simulink model "bettersmcmodel"  (R2015a)
settings: Solver=FixedStepDiscrete  SolverMode=SingleTasking  StartTime=0.0  StopTime=2.5  RelTol=1e-3
PreLoadFcn:
  | Ts_Power=1e-6;
  | Ts_Control=100e-6;
undefined symbols (not defined in the file): D1, Delta, sigbuilder_block
libraries: powerlib x24, powerlib_meascontrol x11, re_lib x1, simulink x1
(part 1 of 2)
Description:
  | Copyright 2008-2015 The MathWorks, Inc.
settings Model: SimulationMode=accelerator  CovSFcnEnable=off  Creator=MathWorks  LastModifiedBy=teja
settings DataIOCC: SignalLoggingSaveFormat=ModelDataLogs  SignalLogging=off  DSMLogging=off
settings OptimizationCC: ExpressionDepthLimit=2147483647
settings DebuggingCC: UnderspecifiedInitializationDetection=Classic  MergeDetectMultiDrivingBlocksExec=none  SolverPrmCheckMsg=warning  FcnCallInpInsideContextMsg=UseLocalSettings  StateNameClashWarn=warning
settings GRTTargetCC: CombineOutputUpdateFcns=off  GRTInterface=on

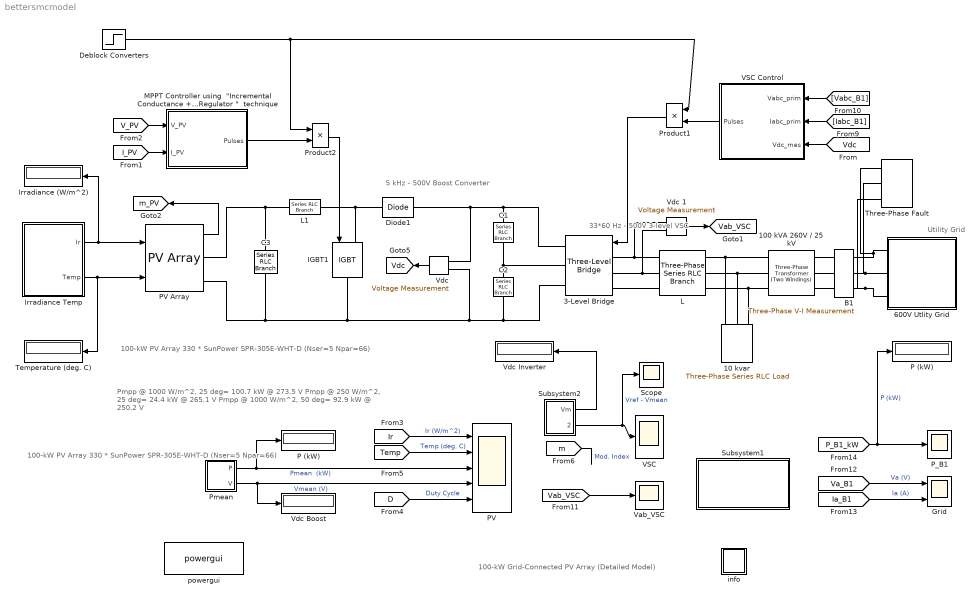
== system bettersmcmodel ==
  note: 5 kHz - 500V
      | Boost Converter
  note: 33*60 Hz - 500V
      | 3-level VSC
  note: 100-kW Grid-Connected PV Array (Detailed Model)
  note: Utility Grid
  note: Pmpp @ 1000 W/m^2, 25 deg= 100.7 kW @ 273.5 V
      | Pmpp @  250 W/m^2, 25 deg= 24.4  kW @ 265.1 V
      | Pmpp @ 1000 W/m^2, 50 deg= 92.9  kW @ 250.2 V
  note: 100-kW  PV Array
      | 330 * SunPower SPR-305E-WHT-D  (Nser=5 Npar=66)
  note: 100-kW  PV Array
      | 330 * SunPower SPR-305E-WHT-D  (Nser=5 Npar=66)
  10 kvar : powerlib/Elements/Three-Phase Series RLC Load  LConnTagsString=A|B|C  Configuration=Y (grounded)  NominalVoltage=240  NominalFrequency=60  ActivePower=10e3/100  InductivePower=0  CapacitivePower=10e3  Measurements=None  LoadType=constant Z
  100 kVA 260V / 25 kV : powerlib/Elements/Three-Phase Transformer (Two Windings)  Winding1Connection=Yg  Winding2Connection=Delta (D1)  CoreType=Three single-phase transformers  SetSaturation=off  Hysteresis=off  DataFile='hysteresis'  SetInitialFlux=off  Measurements=None  UNITS=pu  NominalPower=[100e3 , 60 ]  Winding1=[ 25e3 , 0.001 , 0.03 ]  Winding2=[ 260 , 0.001 , 0.03 ]  Rm=500  Lm=500  L0=0.5  Saturation=[ 0,0 ; 0.0024,1.2 ; 1.0,1.52 ]  InitialFluxes=[ 0.8 , -0.8 , 0.7 ]  MoreParameters=off  BreakLoop=off  DataType=off  TransfoNumber=0
  3-Level Bridge : powerlib/Power Electronics/Three-Level Bridge  Arms=3  SnubberResistance=1e6  SbubberCapacitance=inf  Device=IGBT / Diodes  Ron=0.2e-3  ForwardVoltages="[  0  0 ]"  Measurements=None
  600V Utlity Grid : Subsystem
      mask Display: image(imread('grid.jpg'))
  B1 : powerlib/Measurements/Three-Phase V-I Measurement  VoltageMeasurement=phase-to-ground  SetLabelV=on  LabelV=Vabc_B1  Vpu=off  VpuLL=off  CurrentMeasurement=yes  SetLabelI=on  LabelI=Iabc_B1  Ipu=off  Pbase=100e6  Vbase=500e3  OutputType=Magnitude  PhasorSimulation=off  PSBequivalent=0
  C1 : powerlib/Elements/Series RLC Branch  LConnTagsString=__new0  RConnTagsString=__new0  BranchType=C  Resistance=1.0  Inductance=1.0  SetiL0=off  InitialCurrent=0  Capacitance=12000e-06  Setx0=off  InitialVoltage=0  Measurements=None
  C2 : powerlib/Elements/Series RLC Branch  LConnTagsString=__new0  RConnTagsString=__new0  BranchType=C  Resistance=1.0  Inductance=1.0  SetiL0=off  InitialCurrent=0  Capacitance=12000e-06  Setx0=off  InitialVoltage=0  Measurements=None
  C3 : powerlib/Elements/Series RLC Branch  LConnTagsString=__new0  RConnTagsString=__new0  BranchType=C  Resistance=1.0  Inductance=1.0  SetiL0=off  InitialCurrent=0  Capacitance=100e-6  Setx0=off  InitialVoltage=0  Measurements=Branch voltage
  Deblock Converters : Step  Time=0.05  SampleTime=0
  Diode1 : powerlib/Power Electronics/Diode  Ron=1e-4  Lon=0  Vf=0  IC=0  UseSnubber=off  Rs=inf  Cs=inf  Measurements=off
  Grid : Scope  NumInputPorts=2
      settings: TimeRange=0.05  YMin=-15000~-2.5  YMax=15000~4  Decimation=20
  IGBT1 : powerlib/Power Electronics/IGBT  Ron=0.001  Lon=0  Vf=0  Tf=0  Tt=0  IC=0  Rs=1e5  Cs=inf  Measurements=off
  Irradiance (W/m^2) : Display
      settings: Format=bank  Decimation=1000
  Irradiance Temp : Subsystem  Tag=STV Subsys  LoadFcn=sigbuilder_block('load');  StartFcn=sigbuilder_block('start');  StopFcn=sigbuilder_block('stop');  ClipboardFcn=sigbuilder_block('clipboard');  mask(Sigbuilder block){}
      mask help: Sigbuilder GUI
      mask init:
      | if ~strcmp(get_param(bdroot(gcbh),'SimulationStatus'),'stopped') tuvar = sigbuilder_block('maskInit'); end
      settings: CopyFcn=sigbuilder_block('copy');  DeleteFcn=sigbuilder_block('delete');  ModelCloseFcn=sigbuilder_block('modelClose');  PreSaveFcn=sigbuilder_block('preSave');  PauseFcn=sigbuilder_block('pause')  ContinueFcn=sigbuilder_block('continue')  NameChangeFcn=sigbuilder_block('namechange');  OpenFcn=sigbuilder_block('open',[216.75 153.75 550.5 395.25 ]);  CloseFcn=sigbuilder_block('close');
      mask Display: plot(0,0,100,100,[10,10,40,40,10],[80,20,20,80,80],[40,10],[50,50], [40,27,10],[65,72,56],[40,25,25,10],[28,28,43,43]);
  L : powerlib/Elements/Three-Phase Series RLC Branch  LConnTagsString=A|B|C  RConnTagsString=A|B|C  BranchType=RL  Resistance=500e-6*377/50/2  Inductance=500e-6/2  Capacitance=inf  Measurements=None
  L1 : powerlib/Elements/Series RLC Branch  LConnTagsString=__new0  RConnTagsString=__new0  BranchType=RL  Resistance=0.005  Inductance=5e-3  SetiL0=off  InitialCurrent=0  Capacitance=1e-6  Setx0=off  InitialVoltage=0  Measurements=None
  "MPPT Controller using  \"Incremental Conductance + Integral Regulator \"  technique " : Subsystem  mask(Boost Control - MPPT){fc=5000, T_MPPT=200e-6, Dinit=0.5}
      mask prompts: fc "PWM switching frequency (Hz)"; T_MPPT "Time window used by MPPT control (s)"; Dinit "Initial value of duty cycle"
  P (kW) : Display
      settings: Format=bank  Decimation=2000
  "P (kW) " : Display
      settings: Format=bank  Decimation=2000
  PV : Scope  NumInputPorts=5
      settings: TimeRange=2.5  YMin=200~25~0~0~0.44  YMax=1000~50~150~400~0.52  Decimation=100
  PV Array : re_lib/Solar/PV Array  Npar=66  Nser=5  PlotType=array @ 1000 W/m2 & specified temperatures  S_vec="[ 1000  250 ]"  Temp_C_vec="[0 25 50  ]"  ModuleName=SunPower SPR-305E-WHT-D  PlotWhenSelected=off  Pm=305.226  Ncell=96  Voc=64.2  Isc=5.96  Vm=54.7  Im=5.58  beta_Voc_pc=-0.27269  alpha_Isc_pc=0.061745  beta_Voc=-0.17507  alpha_Isc=0.00368  IL=6.0092  I0=6.3014e-12  nI=0.94504  Rsh=269.5934  Rs=0.37152  BAL=on  Tc=Tc  Tfilter=5e-5
  P_B1 : Scope
      settings: TimeRange=2  YMin=50.4558  YMax=55.767  SaveName=c3  Decimation=100
  Pmean : Subsystem
  Product1 : Product  RndMeth=Zero
  Product2 : Product  RndMeth=Zero
  Scope : Scope
      settings: SaveName=c2
  Subsystem1 : Subsystem
      mask Display: disp('Open this block\nto display additional \nscopes & measurements')
  Subsystem2 : Subsystem
  "Temperature (deg. C)\t" : Display
      settings: Format=bank  Decimation=1000
  Three-Phase Fault : powerlib/Elements/Three-Phase Fault  InitialStates=0  FaultA=on  FaultB=on  FaultC=on  GroundFault=on  SwitchTimes="[1/60  5/60]"  External=off  SwitchStatus=NaN  FaultResistance=0.001  GroundResistance=0.01  SnubberResistance=1e6  SnubberCapacitance=inf  Measurements=None
  VSC : Scope
      settings: TimeRange=2  YMin=500  YMax=590  SaveName=S  Decimation=100
  VSC Control : Subsystem  mask(VSC Main Controller){nom=[ 100e3  60 ], Vnom=[ 25e3 260 ], Vnom_dc=500, RLxfo=[0.002  0.06 ], RLchoke=[2e-3  250e-6  ], K_VDCreg=[7  800], K_Ireg=[0.3 20], Ts=Ts_Control}
      mask prompts: nom "Nominal power and frequency [ Pnom(VA)  Fnom(Hz) ]:"; Vnom "Nominal primary and secondary voltages (Vrms LL) [ Vnom_prim   Vnom_sec ]:"; Vnom_dc "Nominal DC bus voltage (V):"; RLxfo "Total transformer leakage impedance (pu/Pnom) [ Rxfo  Lxf ]"; RLchoke "Choke impedance [ R(ohm) L(H) ]"; K_VDCreg "VDC regultator gains [ Kp  Ki ]:"; K_Ireg "Current regulator gains [ Kp  Ki ]:"; Ts "Sample time"
      mask init:
      | Pnom=nom(1);
      | Fnom=nom(2);
      | Vnom_prim=Vnom(1);
      | Vnom_sec=Vnom(2);
      | Zbase=Vnom_sec^2/Pnom;
      | Rtot_pu=RLxfo(1) + RLchoke(1)/Zbase;
      | Ltot_pu=RLxfo(2) + RLchoke(2)/(Zbase/(2*pi*Fnom));
      | Kp_VDCreg=K_VDCreg(1);
      | Ki_VDCreg=K_VDCreg(2);
      | Kp_Ireg=K_Ireg(1);
      | Ki_Ireg=K_Ireg(2);
      | Vdc_ref=Vnom_dc;
      | % Used to determine initial value of Boost Control (MPPT)
      | assignin('base','Vdc_ref_Inv',Vdc_ref);
  Vab_VSC : Scope
      settings: TimeRange=2  SaveName=c1  Decimation=10
  "Vdc " : powerlib/Measurements/Voltage Measurement  Tag=PoWeRsYsTeMmEaSuReMeNt  PhasorSimulation=off  OutputType=Magnitude  PSBequivalent=0
  Vdc 1 : powerlib/Measurements/Voltage Measurement  Tag=PoWeRsYsTeMmEaSuReMeNt  PhasorSimulation=off  OutputType=Magnitude  PSBequivalent=0
  Vdc Boost : Display
      settings: Format=bank  Decimation=2000
  Vdc Inverter : Display
      settings: Format=bank  Decimation=2000
  info : Subsystem
      settings: OpenFcn=showdemo(bdroot(gcb))
      mask Display: disp('?')
  powergui : powerlib/powergui  Priority=1  SimulationMode=Discrete  SolverType=Tustin/Backward Euler (TBE)  SampleTime=Ts_Power  frequency=60  SPID=off  DisableSnubberDevices=off  DisableRonSwitches=off  DisableVfSwitches=off  SwTol=0  DisplayEquations=off  Interpol=off  methode=off  Ts=0  FunctionMessages=off  echomessages=off  HookPort=off  EnableUseOfTLC=off  x0status=blocks  frequencyindice=0  Pbase=100e6  ErrMax=1e-4  Iterations=50  UnitsV=kV  UnitsW=MW  buscounter=0  RestoreLinks=warning  ResistiveCurrentMeasurement=off  Frange=[0:2:500]  Ylog=off  Xlog=on  ShowGrid=off  save=off  variable=ZData  structure=0  ZoomFFT=on  StartTime=0.0  cycles=1  DisplayStyle=1  fundamental=60  FreqAxis=off  MaxFrequency=1000  frequencyindicesteady=1  RmsSteady=1  display=off
  tag scope: Vab_VSC=global, Vdc=global, m_PV=global
  wires:
  "Vdc "/1 -> [Vdc]
  Product2/1 -> IGBT1/1
  "MPPT Controller using  \"Incremental Conductance + Integral Regulator \"  technique "/1(Pulses) -> Product2/2
  Deblock Converters/1 -> Product2/1, Product1/1
  [Vabc_B1] -> VSC Control/1(Vabc_prim)
  [Iabc_B1] -> VSC Control/2(Iabc_prim)
  [Vdc] -> VSC Control/3(Vdc_mes)
  VSC Control/1(Pulses) -> Product1/2
  Product1/1 -> 3-Level Bridge/1
  [I_PV] -> "MPPT Controller using  \"Incremental Conductance + Integral Regulator \"  technique "/2(I_PV)
  [V_PV] -> "MPPT Controller using  \"Incremental Conductance + Integral Regulator \"  technique "/1(V_PV)
  Pmean/1(P) -> "P (kW) "/1, PV/3  "Pmean  (kW)"
  [m] -> ?  "Mod. Index"
  Vdc 1/1 -> [Vab_VSC]
  [Vab_VSC] -> Vab_VSC/1
  [Ia_B1] -> Grid/2  "Ia (A)"
  [Va_B1] -> Grid/1  "Va (V)"
  [P_B1_kW] -> P_B1/1, P (kW)/1  "P (kW)"
  Pmean/2(V) -> Vdc Boost/1, PV/4  "Vmean (V)"
  Subsystem2/2(VrVm) -> Scope/1, VSC/1  "Vref - Vmean"
  Subsystem2/1(Vm) -> Vdc Inverter/1
  PV Array/1 -> [m_PV]
  Irradiance Temp/1(Ir) -> PV Array/1, Irradiance (W/m^2)/1
  Irradiance Temp/2(Temp) -> PV Array/2, "Temperature (deg. C)\t"/1
  [D] -> PV/5  "Duty Cycle"
  [Temp] -> PV/2  "Temp (deg. C)"
  [Ir] -> PV/1  "Ir (W/m^2)"
  connections:
  3-Level Bridge/RConn1 -- Diode1/RConn1 -- "Vdc "/LConn1 -- C1/LConn1
  L1/RConn1 -- Diode1/LConn1 -- IGBT1/LConn1
  3-Level Bridge/RConn3 -- C2/RConn1 -- "Vdc "/LConn2 -- IGBT1/RConn1 -- PV Array/RConn2 -- C3/RConn1
  3-Level Bridge/LConn1 -- L/LConn1 -- Vdc 1/LConn1
  3-Level Bridge/LConn2 -- L/LConn2 -- Vdc 1/LConn2
  3-Level Bridge/LConn3 -- L/LConn3
  L/RConn1 -- 100 kVA 260V / 25 kV/RConn1 -- 10 kvar/LConn1
  L/RConn2 -- 100 kVA 260V / 25 kV/RConn2 -- 10 kvar/LConn2
  L/RConn3 -- 100 kVA 260V / 25 kV/RConn3 -- 10 kvar/LConn3
  B1/LConn1 -- 100 kVA 260V / 25 kV/LConn1
  B1/LConn2 -- 100 kVA 260V / 25 kV/LConn2
  B1/LConn3 -- 100 kVA 260V / 25 kV/LConn3
  C2/LConn1 -- C1/RConn1 -- 3-Level Bridge/RConn2
  C3/LConn1 -- PV Array/RConn1 -- L1/LConn1
  B1/RConn2 -- 600V Utlity Grid/LConn2 -- Three-Phase Fault/LConn2
  B1/RConn1 -- Three-Phase Fault/LConn1 -- 600V Utlity Grid/LConn1
  B1/RConn3 -- 600V Utlity Grid/LConn3 -- Three-Phase Fault/LConn3

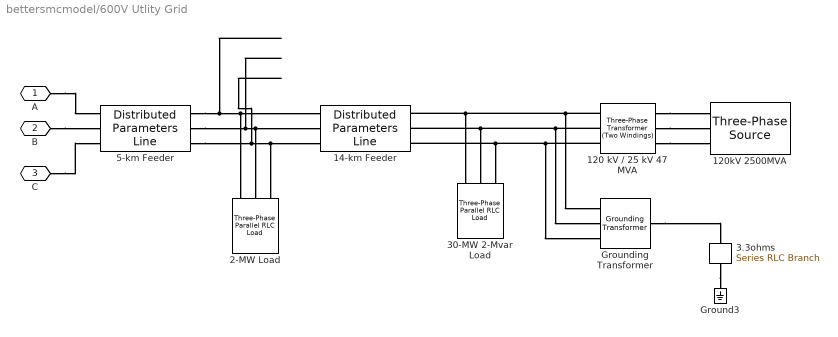
== system bettersmcmodel/600V Utlity Grid ==
  120 kV / 25 kV 47 MVA : powerlib/Elements/Three-Phase Transformer (Two Windings)  Winding1Connection=Yg  Winding2Connection=Delta (D1)  CoreType=Three single-phase transformers  SetSaturation=off  Hysteresis=off  DataFile='basic_model'  SetInitialFlux=off  Measurements=None  UNITS=pu  NominalPower=[47e6 60 ]  Winding1="[ 120e3  0.08/30   0.08 ]"  Winding2="[ 25e3  0.08/30  0.08]"  Rm=500  Lm=500  L0=0.5  Saturation="[ 0,0  ;  0.005,1.2  ;  1.0,1.4 ]"  InitialFluxes=[ 0.8 , -0.8 , 0.7 ]  MoreParameters=off  BreakLoop=off  DataType=off  TransfoNumber=0
  120kV 2500MVA : powerlib/Electrical Sources/Three-Phase Source  Voltage=120e3  PhaseAngle=0  Frequency=60  InternalConnection=Yg  SpecifyImpedance=on  Resistance=0.8929  Inductance=16.58e-3  ShortCircuitLevel=2500e6  BaseVoltage=120e3  XRratio=7  BusType=swing  Pref=0  Qref=0  Qmin=-inf  Qmax=inf
  14-km Feeder : powerlib/Elements/Distributed Parameters Line  Phases=3  Frequency=60  Resistance=[0.1153 0.413]  Inductance=[1.05e-3 3.32e-3]  Capacitance=[11.33e-009 5.01e-009]  Length=14  x1=[-5.8e-05 -2.78846572041482e-09 0 0;-5.7e-05 -2.78728594542614e-09 0 0;-5.6e-05 -2.78610577430196e-09 0 0;-5.5e-05 -2.78492520721002e-09 0 0;-5.4e-05 -2.7837442443181e-09 0 0;-5.3e-05 -2.78256288579404e-09 0 0;-5.2e-05 -2.78138113180574e-09 0 0;-5.1e-05 -2.78019898252115e-09 0 0;-5e-05 -2.77901643810828e-09 0 0;-4.9e-05 -2.7778334987352e-09 -3790.91356131619 -24061.331995883;-4.8e-05 -2.77665016457003e-09 -3781.84238368431 -24062.7594267666;-4.7e-05 -2.77546643578094e-09 -3772.77066856828 -24064.1834377954;-4.6e-05 -2.77428231253618e-09 -3763.6984172574 -24065.6040287671;-4.5e-05 -2.77309779500403e-09 -3754.62563104105 -24067.0211994797;-4.4e-05 -2.77191288335284e-09 -3745.55231120865 -24068.4349497319;-4.3e-05 -2.77072757775101e-09 -3736.47845904974 -24069.8452793227;-4.2e-05 -2.76954187836699e-09 -3727.40407585391 -24071.2521880517;-4.1e-05 -2.76835578536932e-09 -3718.32916291083 -24072.6556757189;-4e-05 -2.76716929892654e-09 -3709.25372151026 -24074.0557421249;-3.9e-05 -2.7659824192073e-09 -3700.177752942 -24075.4523870707;-3.8e-05 -2.76479514638027e-09 -3691.10125849597 -24076.8456103578;-3.7e-05 -2.76360748061418e-09 -3682.02423946214 -24078.2354117881;-3.6e-05 -2.76241942207785e-09 -3672.94669713054 -24079.6217911643;-3.5e-05 -2.7612309709401e-09 -3663.8686327913 -24081.0047482891;-3.4e-05 -2.76004212736986e-09 -3654.79004773462 -24082.3842829662;-3.3e-05 -2.75885289153607e-09 -3645.71094325077 -24083.7603949993;-3.2e-05 -2.75766326360776e-09 -3636.63132063009 -24085.133084193;-3.1e-05 -2.756473243754e-09 -3627.55118116299 -24086.5023503521;-3e-05 -2.75528283214392e-09 -3618.47052613997 -24087.8681932821;-2.9e-05 -2.7540920289467e-09 -3609.38935685159 -24089.2306127888;-2.8e-05 -2.75290083433159e-09 -3600.30767458848 -24090.5896086786;-2.7e-05 -2.75170924846787e-09 -3591.22548064137 -24091.9451807584;-2.6e-05 -2.75051727152489e-09 -3582.14277630102 -24093.2973288354;-2.5e-05 -2.74932490367208e-09 -3573.05956285829 -24094.6460527176;-2.4e-05 -2.74813214507888e-09 -3563.97584160412 -24095.9913522133;-2.3e-05 -2.74693899591481e-09 -3554.8916138295 -24097.3332271312;-2.2e-05 -2.74574545634945e-09 -3545.80688082549 -24098.6716772806;-2.1e-05 -2.74455152655243e-09 -3536.72164388326 -24100.0067024713;-2e-05 -2.74335720669342e-09 -3527.635904294 -24101.3383025136;-1.9e-05 -2.74216249694218e-09 -3518.54966334901 -24102.6664772183;-1.8e-05 -2.74096739746849e-09 -3509.46292233964 -24103.9912263965;-1.7e-05 -2.7397719084422e-09 -3500.37568255732 -24105.31254986;-1.6e-05 -2.73857603003323e-09 -3491.28794529356 -24106.630447421;-1.5e-05 -2.73737976241153e-09 -3482.19971183991 -24107.9449188921;-1.4e-05 -2.73618310574711e-09 -3473.11098348803 -24109.2559640867;-1.3e-05 -2.73498606021005e-09 -3464.02176152962 -24110.5635828183;-1.2e-05 -2.73378862597048e-09 -3454.93204725646 -24111.8677749011;-1.1e-05 -2.73259080319858e-09 -3445.84184196041 -24113.1685401498;-1e-05 -2.73139259206458e-09 -3436.75114693339 -24114.4658783794;-9e-06 -2.73019399273878e-09 -3427.65996346738 -24115.7597894057;-8e-06 -2.72899500539153e-09 -3418.56829285445 -24117.0502730447;-7e-06 -2.72779563019322e-09 -3409.47613638673 -24118.337329113;-6e-06 -2.72659586731433e-09 -3400.38349535641 -24119.6209574276;-5e-06 -2.72539571692535e-09 -3391.29037105576 -24120.9011578063;-4e-06 -2.72419517919685e-09 -3382.19676477711 -24122.1779300669;-3e-06 -2.72299425429947e-09 -3373.10267781288 -24123.4512740281;-2e-06 -2.72179294240388e-09 -3364.00811145553 -24124.7211895088;-1e-06 -2.72059124368081e-09 -3354.91306699761 -24125.9876763287]  x2=[-5.8e-05 -2.84238474455657e-09 0 0;-5.7e-05 -2.8410909495707e-09 0 0;-5.6e-05 -2.83979675080246e-09 0 0;-5.5e-05 -2.83850214843576e-09 0 0;-5.4e-05 -2.8372071426546e-09 0 0;-5.3e-05 -2.83591173364303e-09 0 0;-5.2e-05 -2.83461592158516e-09 0 0;-5.1e-05 -2.83331970666515e-09 0 0;-5e-05 -2.83202308906722e-09 0 0;-4.9e-05 -2.83072606897565e-09 -3379.44571071679 -24244.0324946947;-4.8e-05 -2.82942864657478e-09 -3370.30568586053 -24245.3047928739;-4.7e-05 -2.828130822049e-09 -3361.16518200868 -24246.5736452545;-4.6e-05 -2.82683259558275e-09 -3352.02420046029 -24247.8390516562;-4.5e-05 -2.82553396736055e-09 -3342.8827425145 -24249.1010118993;-4.4e-05 -2.82423493756696e-09 -3333.74080947053 -24250.3595258043;-4.3e-05 -2.8229355063866e-09 -3324.59840262764 -24251.6145931924;-4.2e-05 -2.82163567400415e-09 -3315.45552328517 -24252.8662138852;-4.1e-05 -2.82033544060434e-09 -3306.31217274253 -24254.1143877048;-4e-05 -2.81903480637196e-09 -3297.1683522992 -24255.3591144739;-3.9e-05 -2.81773377149187e-09 -3288.02406325471 -24256.6003940155;-3.8e-05 -2.81643233614897e-09 -3278.87930690867 -24257.8382261532;-3.7e-05 -2.81513050052823e-09 -3269.73408456076 -24259.0726107112;-3.6e-05 -2.81382826481466e-09 -3260.58839751071 -24260.3035475139;-3.5e-05 -2.81252562919334e-09 -3251.44224705834 -24261.5310363864;-3.4e-05 -2.8112225938494e-09 -3242.29563450351 -24262.7550771543;-3.3e-05 -2.80991915896804e-09 -3233.14856114616 -24263.9756696435;-3.2e-05 -2.8086153247345e-09 -3224.0010282863 -24265.1928136808;-3.1e-05 -2.80731109133408e-09 -3214.85303722399 -24266.4065090929;-3e-05 -2.80600645895215e-09 -3205.70458925937 -24267.6167557075;-2.9e-05 -2.80470142777413e-09 -3196.55568569263 -24268.8235533526;-2.8e-05 -2.80339599798548e-09 -3187.40632782404 -24270.0269018566;-2.7e-05 -2.80209016977174e-09 -3178.25651695392 -24271.2268010485;-2.6e-05 -2.8007839433185e-09 -3169.10625438268 -24272.4232507578;-2.5e-05 -2.79947731881139e-09 -3159.95554141076 -24273.6162508144;-2.4e-05 -2.79817029643613e-09 -3150.80437933868 -24274.8058010489;-2.3e-05 -2.79686287637846e-09 -3141.65276946704 -24275.991901292;-2.2e-05 -2.7955550588242e-09 -3132.50071309647 -24277.1745513753;-2.1e-05 -2.79424684395923e-09 -3123.34821152769 -24278.3537511307;-2e-05 -2.79293823196946e-09 -3114.19526606148 -24279.5295003906;-1.9e-05 -2.79162922304088e-09 -3105.04187799866 -24280.7017989878;-1.8e-05 -2.79031981735953e-09 -3095.88804864015 -24281.8706467558;-1.7e-05 -2.7890100151115e-09 -3086.7337792869 -24283.0360435285;-1.6e-05 -2.78769981648295e-09 -3077.57907123994 -24284.1979891402;-1.5e-05 -2.78638922166009e-09 -3068.42392580036 -24285.3564834258;-1.4e-05 -2.78507823082918e-09 -3059.26834426931 -24286.5115262206;-1.3e-05 -2.78376684417654e-09 -3050.112327948 -24287.6631173605;-1.2e-05 -2.78245506188854e-09 -3040.9558781377 -24288.8112566818;-1.1e-05 -2.78114288415163e-09 -3031.79899613976 -24289.9559440214;-1e-05 -2.7798303111523e-09 -3022.64168325557 -24291.0971792165;-9e-06 -2.77851734307708e-09 -3013.48394078658 -24292.234962105;-8e-06 -2.77720398011258e-09 -3004.32577003432 -24293.3692925251;-7e-06 -2.77589022244546e-09 -2995.16717230036 -24294.5001703157;-6e-06 -2.77457607026243e-09 -2986.00814888636 -24295.627595316;-5e-06 -2.77326152375026e-09 -2976.848701094 -24296.7515673657;-4e-06 -2.77194658309578e-09 -2967.68883022505 -24297.8720863053;-3e-06 -2.77063124848587e-09 -2958.52853758134 -24298.9891519753;-2e-06 -2.76931552010748e-09 -2949.36782446474 -24300.102764217;-1e-06 -2.76799939814759e-09 -2940.20669217719 -24301.2129228722]  x3=[-5.8e-05 -2.00460551784577e-11 0 0;-5.7e-05 -2.00435398524558e-11 0 0;-5.6e-05 -2.00410216778199e-11 0 0;-5.5e-05 -2.00385006549079e-11 0 0;-5.4e-05 -2.0035976784078e-11 0 0;-5.3e-05 -2.00334500656889e-11 0 0;-5.2e-05 -2.00309205000999e-11 0 0;-5.1e-05 -2.00283880876703e-11 0 0;-5e-05 -2.00258528287601e-11 0 0;-4.9e-05 -2.00233147237296e-11 -23.5492221256945 -155.70495879038;-4.8e-05 -2.00207737729395e-11 -23.4905210670905 -155.713825573184;-4.7e-05 -2.0018229976751e-11 -23.4318166699595 -155.72267022558;-4.6e-05 -2.00156833355256e-11 -23.3731089426448 -155.731492746312;-4.5e-05 -2.00131338496251e-11 -23.3143978934901 -155.740293134126;-4.4e-05 -2.00105815194121e-11 -23.2556835308395 -155.74907138777;-4.3e-05 -2.00080263452491e-11 -23.1969658630377 -155.757827505999;-4.2e-05 -2.00054683274993e-11 -23.1382448984296 -155.766561487566;-4.1e-05 -2.00029074665264e-11 -23.0795206453609 -155.775273331231;-4e-05 -2.00003437626942e-11 -23.0207931121777 -155.783963035756;-3.9e-05 -1.99977772163671e-11 -22.9620623072263 -155.792630599905;-3.8e-05 -1.99952078279099e-11 -22.9033282388538 -155.801276022447;-3.7e-05 -1.99926355976878e-11 -22.8445909154075 -155.809899302153;-3.6e-05 -1.99900605260662e-11 -22.7858503452354 -155.818500437797;-3.5e-05 -1.99874826134112e-11 -22.7271065366859 -155.827079428158;-3.4e-05 -1.99849018600892e-11 -22.6683594981076 -155.835636272015;-3.3e-05 -1.9982318266467e-11 -22.6096092378499 -155.844170968154;-3.2e-05 -1.99797318329117e-11 -22.5508557642625 -155.852683515359;-3.1e-05 -1.99771425597909e-11 -22.4920990856955 -155.861173912423;-3e-05 -1.99745504474726e-11 -22.4333392104997 -155.869642158138;-2.9e-05 -1.99719554963252e-11 -22.3745761470261 -155.878088251301;-2.8e-05 -1.99693577067176e-11 -22.3158099036262 -155.886512190711;-2.7e-05 -1.99667570790189e-11 -22.257040488652 -155.894913975171;-2.6e-05 -1.99641536135987e-11 -22.1982679104561 -155.903293603487;-2.5e-05 -1.9961547310827e-11 -22.1394921773911 -155.911651074468;-2.4e-05 -1.99589381710743e-11 -22.0807132978106 -155.919986386926;-2.3e-05 -1.99563261947114e-11 -22.0219312800683 -155.928299539677;-2.2e-05 -1.99537113821094e-11 -21.9631461325185 -155.936590531539;-2.1e-05 -1.99510937336401e-11 -21.9043578635158 -155.944859361334;-2e-05 -1.99484732496754e-11 -21.8455664814153 -155.953106027887;-1.9e-05 -1.99458499305877e-11 -21.7867719945726 -155.961330530025;-1.8e-05 -1.994322377675e-11 -21.7279744113437 -155.96953286658;-1.7e-05 -1.99405947885354e-11 -21.6691737400851 -155.977713036386;-1.6e-05 -1.99379629663175e-11 -21.6103699891537 -155.985871038281;-1.5e-05 -1.99353283104705e-11 -21.5515631669067 -155.994006871104;-1.4e-05 -1.99326908213687e-11 -21.492753281702 -156.0021205337;-1.3e-05 -1.99300504993871e-11 -21.4339403418977 -156.010212024916;-1.2e-05 -1.99274073449007e-11 -21.3751243558524 -156.018281343601;-1.1e-05 -1.99247613582854e-11 -21.3163053319253 -156.026328488609;-1e-05 -1.99221125399172e-11 -21.2574832784758 -156.034353458796;-9e-06 -1.99194608901724e-11 -21.1986582038639 -156.042356253022;-8e-06 -1.9916806409428e-11 -21.1398301164499 -156.050336870149;-7e-06 -1.99141490980613e-11 -21.0809990245945 -156.058295309043;-6e-06 -1.99114889564498e-11 -21.0221649366591 -156.066231568572;-5e-06 -1.99088259849717e-11 -20.9633278610051 -156.07414564761;-4e-06 -1.99061601840055e-11 -20.9044878059948 -156.08203754503;-3e-06 -1.99034915539299e-11 -20.8456447799906 -156.089907259713;-2e-06 -1.99008200951243e-11 -20.7867987913553 -156.097754790538;-1e-06 -1.98981458079683e-11 -20.7279498484524 -156.105580136391]  x4=[-5.8e-05 1.32145554520631e-11 0 0;-5.7e-05 1.32154032927262e-11 0 0;-5.6e-05 1.32162492551857e-11 0 0;-5.5e-05 1.32170933393215e-11 0 0;-5.4e-05 1.32179355450135e-11 0 0;-5.3e-05 1.32187758721422e-11 0 0;-5.2e-05 1.32196143205879e-11 0 0;-5.1e-05 1.32204508902317e-11 0 0;-5e-05 1.32212855809546e-11 0 0;-4.9e-05 1.32221183926379e-11 -1.35163069912945 -2.12916945889706;-4.8e-05 1.32229493251633e-11 -1.35082792512439 -2.12967886035273;-4.7e-05 1.32237783784127e-11 -1.35002495913656 -2.13018795913354;-4.6e-05 1.32246055522683e-11 -1.34922180128007 -2.13069675516714;-4.5e-05 1.32254308466125e-11 -1.34841845166907 -2.13120524838121;-4.4e-05 1.32262542613281e-11 -1.34761491041774 -2.13171343870348;-4.3e-05 1.32270757962979e-11 -1.34681117764028 -2.13222132606173;-4.2e-05 1.32278954514053e-11 -1.34600725345092 -2.13272891038378;-4.1e-05 1.32287132265338e-11 -1.3452031379639 -2.13323619159748;-4e-05 1.3229529121567e-11 -1.34439883129352 -2.13374316963075;-3.9e-05 1.32303431363892e-11 -1.34359433355408 -2.13424984441153;-3.8e-05 1.32311552708845e-11 -1.34278964485992 -2.13475621586781;-3.7e-05 1.32319655249376e-11 -1.34198476532541 -2.13526228392762;-3.6e-05 1.32327738984333e-11 -1.34117969506494 -2.13576804851904;-3.5e-05 1.32335803912567e-11 -1.34037443419291 -2.13627350957019;-3.4e-05 1.32343850032932e-11 -1.33956898282379 -2.13677866700923;-3.3e-05 1.32351877344284e-11 -1.33876334107205 -2.13728352076437;-3.2e-05 1.32359885845483e-11 -1.33795750905217 -2.13778807076386;-3.1e-05 1.3236787553539e-11 -1.33715148687869 -2.13829231693598;-3e-05 1.32375846412871e-11 -1.33634527466617 -2.13879625920908;-2.9e-05 1.32383798476791e-11 -1.33553887252918 -2.13929989751153;-2.8e-05 1.32391731726021e-11 -1.33473228058233 -2.13980323177176;-2.7e-05 1.32399646159433e-11 -1.33392549894026 -2.14030626191823;-2.6e-05 1.32407541775903e-11 -1.33311852771763 -2.14080898787944;-2.5e-05 1.32415418574309e-11 -1.33231136702912 -2.14131140958395;-2.4e-05 1.3242327655353e-11 -1.33150401698945 -2.14181352696036;-2.3e-05 1.3243111571245e-11 -1.33069647771337 -2.1423153399373;-2.2e-05 1.32438936049956e-11 -1.32988874931564 -2.14281684844345;-2.1e-05 1.32446737564935e-11 -1.32908083191107 -2.14331805240754;-2e-05 1.32454520256279e-11 -1.32827272561446 -2.14381895175833;-1.9e-05 1.32462284122881e-11 -1.32746443054068 -2.14431954642464;-1.8e-05 1.32470029163639e-11 -1.3266559468046 -2.14481983633532;-1.7e-05 1.32477755377452e-11 -1.32584727452112 -2.14531982141927;-1.6e-05 1.3248546276322e-11 -1.32503841380517 -2.14581950160543;-1.5e-05 1.3249315131985e-11 -1.32422936477172 -2.14631887682278;-1.4e-05 1.32500821046249e-11 -1.32342012753574 -2.14681794700035;-1.3e-05 1.32508471941325e-11 -1.32261070221225 -2.14731671206722;-1.2e-05 1.32516104003993e-11 -1.32180108891627 -2.14781517195249;-1.1e-05 1.32523717233167e-11 -1.32099128776289 -2.14831332658532;-1e-05 1.32531311627765e-11 -1.32018129886718 -2.14881117589492;-9e-06 1.32538887186708e-11 -1.31937112234427 -2.14930871981053;-8e-06 1.3254644390892e-11 -1.3185607583093 -2.14980595826144;-7e-06 1.32553981793326e-11 -1.31775020687744 -2.15030289117698;-6e-06 1.32561500838854e-11 -1.31693946816388 -2.15079951848652;-5e-06 1.32569001044438e-11 -1.31612854228386 -2.15129584011948;-4e-06 1.32576482409009e-11 -1.31531742935262 -2.15179185600533;-3e-06 1.32583944931506e-11 -1.31450612948544 -2.15228756607356;-2e-06 1.32591388610867e-11 -1.31369464279762 -2.15278297025373;-1e-06 1.32598813446035e-11 -1.31288296940449 -2.15327806847543]  x5=5.70973484498186e-05  V1=ones(3,3)  V2=ones(3,3)  I1=ones(3,3)  I2=ones(3,3)  nHarmo=1  Measurements=None
  2-MW Load : powerlib/Elements/Three-Phase Parallel RLC Load  LConnTagsString=A|B|C  Configuration=Y (grounded)  NominalVoltage=25e3  NominalFrequency=60  ActivePower=2e6  InductivePower=0  CapacitivePower=0  Measurements=None  LoadType=constant Z
  "3.3ohms " : powerlib/Elements/Series RLC Branch  LConnTagsString=__new0  RConnTagsString=__new0  BranchType=R  Resistance=3.3  Inductance=[]  SetiL0=off  InitialCurrent=0  Capacitance=[]  Setx0=off  InitialVoltage=0  Measurements=None
  30-MW 2-Mvar Load : powerlib/Elements/Three-Phase Parallel RLC Load  LConnTagsString=A|B|C  Configuration=Y (grounded)  NominalVoltage=25e3  NominalFrequency=60  ActivePower=30e6  InductivePower=2e6  CapacitivePower=0  Measurements=None  LoadType=constant Z
  5-km Feeder : powerlib/Elements/Distributed Parameters Line  Phases=3  Frequency=60  Resistance=[0.1153 0.413]  Inductance=[1.05e-3 3.32e-3]  Capacitance=[11.33e-009 5.01e-009]  Length=5  x1=[-2.1e-05 -2.68247201757925e-09 -3537.40246322704 -24101.3113737726;-2e-05 -2.68128874623808e-09 -3528.31623173992 -24102.643230385;-1.9e-05 -2.68010509382599e-09 -3519.22949880037 -24103.9716614744;-1.8e-05 -2.67892106051119e-09 -3510.14226569983 -24105.2966668517;-1.7e-05 -2.67773664646197e-09 -3501.0545337298 -24106.6182463289;-1.6e-05 -2.67655185184664e-09 -3491.96630418183 -24107.9363997179;-1.5e-05 -2.67536667683361e-09 -3482.87757834758 -24109.2511268316;-1.4e-05 -2.67418112159131e-09 -3473.78835751874 -24110.5624274829;-1.3e-05 -2.67299518628823e-09 -3464.69864298711 -24111.8703014857;-1.2e-05 -2.67180887109293e-09 -3455.60843604454 -24113.174748654;-1.1e-05 -2.670622176174e-09 -3446.51773798294 -24114.4757688023;-1e-05 -2.66943510170009e-09 -3437.4265500943 -24115.7733617459;-9e-06 -2.66824764783993e-09 -3428.3348736707 -24117.0675273002;-8e-06 -2.66705981476227e-09 -3419.24271000425 -24118.3582652814;-7e-06 -2.66587160263593e-09 -3410.15006038715 -24119.645575506;-6e-06 -2.66468301162978e-09 -3401.05692611168 -24120.9294577911;-5e-06 -2.66349404191275e-09 -3391.96330847017 -24122.2099119541;-4e-06 -2.66230469365381e-09 -3382.86920875503 -24123.4869378132;-3e-06 -2.661114967022e-09 -3373.77462825873 -24124.7605351867;-2e-06 -2.65992486218641e-09 -3364.67956827382 -24126.0307038938;-1e-06 -2.65873437931618e-09 -3355.5840300929 -24127.2974437538]  x2=[-2.1e-05 -2.74455152655243e-09 -3536.72164388326 -24100.0067024713;-2e-05 -2.74335720669342e-09 -3527.635904294 -24101.3383025136;-1.9e-05 -2.74216249694218e-09 -3518.54966334901 -24102.6664772183;-1.8e-05 -2.74096739746849e-09 -3509.46292233964 -24103.9912263965;-1.7e-05 -2.7397719084422e-09 -3500.37568255732 -24105.31254986;-1.6e-05 -2.73857603003323e-09 -3491.28794529356 -24106.630447421;-1.5e-05 -2.73737976241153e-09 -3482.19971183991 -24107.9449188921;-1.4e-05 -2.73618310574711e-09 -3473.11098348803 -24109.2559640867;-1.3e-05 -2.73498606021005e-09 -3464.02176152962 -24110.5635828183;-1.2e-05 -2.73378862597048e-09 -3454.93204725646 -24111.8677749011;-1.1e-05 -2.73259080319858e-09 -3445.84184196041 -24113.1685401498;-1e-05 -2.73139259206458e-09 -3436.75114693339 -24114.4658783794;-9e-06 -2.73019399273878e-09 -3427.65996346738 -24115.7597894057;-8e-06 -2.72899500539153e-09 -3418.56829285445 -24117.0502730447;-7e-06 -2.72779563019322e-09 -3409.47613638673 -24118.337329113;-6e-06 -2.72659586731433e-09 -3400.38349535641 -24119.6209574276;-5e-06 -2.72539571692535e-09 -3391.29037105576 -24120.9011578063;-4e-06 -2.72419517919685e-09 -3382.19676477711 -24122.1779300669;-3e-06 -2.72299425429947e-09 -3373.10267781288 -24123.4512740281;-2e-06 -2.72179294240388e-09 -3364.00811145553 -24124.7211895088;-1e-06 -2.72059124368081e-09 -3354.91306699761 -24125.9876763287]  x3=[-2.1e-05 -1.04786200744822e-11 -11.1612525032937 -79.1599286966311;-2e-05 -1.0479443852297e-11 -11.1314091208149 -79.1641307644001;-1.9e-05 -1.04802661407491e-11 -11.1015641563146 -79.1683215811806;-1.8e-05 -1.04810869397217e-11 -11.0717176140345 -79.172501146377;-1.7e-05 -1.04819062490981e-11 -11.0418694982163 -79.1766694593954;-1.6e-05 -1.04827240687619e-11 -11.0120198131023 -79.1808265196432;-1.5e-05 -1.04835403985968e-11 -10.9821685629346 -79.1849723265298;-1.4e-05 -1.04843552384868e-11 -10.9523157519559 -79.1891068794658;-1.3e-05 -1.0485168588316e-11 -10.9224613844088 -79.1932301778636;-1.2e-05 -1.0485980447969e-11 -10.8926054645364 -79.1973422211373;-1.1e-05 -1.04867908173304e-11 -10.8627479965819 -79.2014430087025;-1e-05 -1.04875996962848e-11 -10.8328889847886 -79.2055325399762;-9e-06 -1.04884070847175e-11 -10.8030284334001 -79.2096108143774;-8e-06 -1.04892129825136e-11 -10.7731663466605 -79.2136778313264;-7e-06 -1.04900173895586e-11 -10.7433027288136 -79.2177335902451;-6e-06 -1.04908203057382e-11 -10.7134375841038 -79.2217780905573;-5e-06 -1.04916217309383e-11 -10.6835709167756 -79.225811331688;-4e-06 -1.0492421665045e-11 -10.6537027310737 -79.229833313064;-3e-06 -1.04932201079445e-11 -10.623833031243 -79.2338440341137;-2e-06 -1.04940170595234e-11 -10.5939618215288 -79.2378434942672;-1e-06 -1.04948125196685e-11 -10.5640891061763 -79.2418316929559]  x4=[-2.1e-05 2.85363616208783e-12 -12.5576818000087 -78.8757309228839;-2e-05 2.85799162049611e-12 -12.5279454583321 -78.8804594522782;-1.9e-05 2.86234667272004e-12 -12.498207336155 -78.8851767710001;-1.8e-05 2.86670131814068e-12 -12.4684674377039 -78.8898828783791;-1.7e-05 2.87105555613913e-12 -12.4387257672055 -78.8945777737463;-1.6e-05 2.87540938609655e-12 -12.4089823288868 -78.8992614564346;-1.5e-05 2.87976280739418e-12 -12.379237126975 -78.9039339257782;-1.4e-05 2.88411581941328e-12 -12.3494901656974 -78.9085951811132;-1.3e-05 2.88846842153521e-12 -12.319741449282 -78.9132452217769;-1.2e-05 2.89282061314136e-12 -12.2899909819565 -78.9178840471086;-1.1e-05 2.89717239361318e-12 -12.2602387679492 -78.922511656449;-1e-05 2.90152376233219e-12 -12.2304848114885 -78.9271280491404;-9e-06 2.90587471867997e-12 -12.2007291168032 -78.9317332245267;-8e-06 2.91022526203815e-12 -12.1709716881222 -78.9363271819533;-7e-06 2.91457539178841e-12 -12.1412125296747 -78.9409099207675;-6e-06 2.91892510731251e-12 -12.1114516456901 -78.9454814403178;-5e-06 2.92327440799225e-12 -12.0816890403981 -78.9500417399546;-4e-06 2.92762329320951e-12 -12.0519247180287 -78.9545908190298;-3e-06 2.9319717623462e-12 -12.022158682812 -78.9591286768968;-2e-06 2.93631981478432e-12 -11.9923909389784 -78.9636553129107;-1e-06 2.94066744990591e-12 -11.9626214907586 -78.9681707264281]  x5=2.03919101606495e-05  V1=ones(3,3)  V2=ones(3,3)  I1=ones(3,3)  I2=ones(3,3)  nHarmo=1  Measurements=None
  Ground3 : powerlib/Elements/Ground  LConnTagsString=a
  "Grounding Transformer " : powerlib/Elements/Grounding Transformer   UNITS=pu  NominalPower="[100e6   60]"  NominalVoltage=25e3  ZeroSequenceImpedance_pu=[0.025 0.75]  MagnetizationBranch_pu=[500 500]  ZeroSequenceImpedance_SI=[0.052083 589.05]  MagnetizationBranch_SI=[1041.7 3.927e+005]  Measurements=None
  A : PMIOPort  Port=1  Side=Left
  B : PMIOPort  Port=2  Side=Left
  C : PMIOPort  Port=3  Side=Left
  connections:
  "3.3ohms "/RConn1 -- Ground3/LConn1
  120 kV / 25 kV 47 MVA/LConn1 -- 120kV 2500MVA/RConn1
  120 kV / 25 kV 47 MVA/LConn2 -- 120kV 2500MVA/RConn2
  120 kV / 25 kV 47 MVA/LConn3 -- 120kV 2500MVA/RConn3
  120 kV / 25 kV 47 MVA/RConn1 -- "Grounding Transformer "/LConn1 -- 14-km Feeder/RConn1 -- 30-MW 2-Mvar Load/LConn1
  120 kV / 25 kV 47 MVA/RConn2 -- "Grounding Transformer "/LConn2 -- 14-km Feeder/RConn2 -- 30-MW 2-Mvar Load/LConn2
  120 kV / 25 kV 47 MVA/RConn3 -- "Grounding Transformer "/LConn3 -- 14-km Feeder/RConn3 -- 30-MW 2-Mvar Load/LConn3
  5-km Feeder/RConn1 -- 14-km Feeder/LConn1 -- 2-MW Load/LConn1
  5-km Feeder/RConn2 -- 14-km Feeder/LConn2 -- 2-MW Load/LConn2
  5-km Feeder/RConn3 -- 14-km Feeder/LConn3 -- 2-MW Load/LConn3
  A/RConn1 -- 5-km Feeder/LConn1
  B/RConn1 -- 5-km Feeder/LConn2
  C/RConn1 -- 5-km Feeder/LConn3
  "Grounding Transformer "/RConn1 -- "3.3ohms "/LConn1

== system bettersmcmodel/Irradiance Temp ==
  Demux : Demux  Tag=STV Demux  Outputs=2
  FromWs : FromWorkspace  Tag=STV FromWs  VariableName=tuvar  SampleTime=0
      SigBuilderData=|
      | common.afterFinalStr = 'Extrapolate'
      | common.sampleTime = '0'
      | dataSet(1).timeRange = [0 1]
      | dataSet(1).name = 'Constant Irradiance'
      | dataSet(2).timeRange = [0 1]
      | dataSet(2).name = 'Step Irradiance'
      | dataSet(3).timeRange = [0 3]
      | dataSet(3).name = 'Ramp-up/down Irradiance'
      | sbobj.Groups(1).Name = 'Constant Irradiance'
      | sbobj.Groups(1).Signals(1).Name = 'Ir'
      | sbobj.Groups(1).Signals(1).XData = [0 1]
      | sbobj.Groups(1).Signals(1).YData = [1000 1000]
      | sbobj.Groups(1).Signals(2).Name = 'Temp'
      | sbobj.Groups(1).Signals(2).XData = [0 1 1 2]
      | sbobj.Groups(1).Signals(2).YData = [0 0 1 1]
      | sbobj.Groups(1).TimeRange = [0 1]
      | sbobj.Groups(2).Name = 'Step Irradiance'
      | sbobj.Groups(2).Signals(1).Name = 'Ir'
      | sbobj.Groups(2).Signals(1).XData = [0 0.252 0.252 1]
      | sbobj.Groups(2).Signals(1).YData = [600 600 1000 1000]
      | sbobj.Groups(2).Signals(2).Name = 'Temp'
      | sbobj.Groups(2).Signals(2).XData = [0 1 1 2]
      | sbobj.Groups(2).Signals(2).YData = [0 0 1 1]
      | sbobj.Groups(2).TimeRange = [0 1]
      | sbobj.Groups(3).Name = 'Ramp-up/down Irradiance'
      | sbobj.Groups(3).Signals(1).Name = 'Ir'
      | sbobj.Groups(3).Signals(1).XData = [0 0.6 1.1 1.2 1.7 3]
      | sbobj.Groups(3).Signals(1).YData = [1000 1000 1000 1000 1000 1000]
      | sbobj.Groups(3).Signals(2).Name = 'Temp'
      | sbobj.Groups(3).Signals(2).XData = [0 1 1.5 2.1 3]
      | sbobj.Groups(3).Signals(2).YData = [25 25 50 50 50]
      | sbobj.Groups(3).TimeRange = [0 3]
  Ir : Outport  Tag=STV Outport
  Temp : Outport  Tag=STV Outport  Port=2
  wires:
  Demux/1 -> Ir/1
  FromWs/1 -> Demux/1
  Demux/2 -> Temp/1

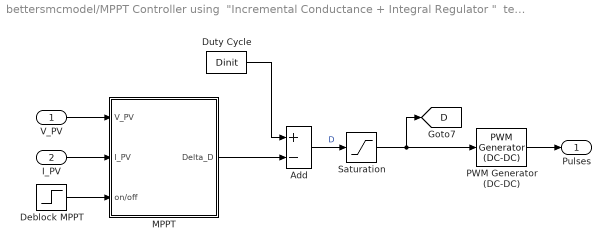
== system bettersmcmodel/MPPT Controller using  "Incremental Conductance + Integral Regulator "  technique  ==
  V_PV : Inport
  I_PV : Inport  Port=2
  Add : Sum  Inputs=+-
  Deblock MPPT : Step  Time=0.4  SampleTime=0
  Duty Cycle : Constant  Value=Dinit
  MPPT : Subsystem
  PWM Generator (DC-DC) : powerlib_meascontrol/Pulse & Signal Generators/PWM Generator (DC-DC)  Fsw=fc  Ts=Ts_Power
  Saturation : Saturate  UpperLimit=1  LowerLimit=0
  Pulses : Outport
  tag scope: D=global
  wires:
  V_PV/1 -> MPPT/1(V_PV)
  I_PV/1 -> MPPT/2(I_PV)
  PWM Generator (DC-DC)/1 -> Pulses/1
  Deblock MPPT/1 -> MPPT/3(on/off)
  Saturation/1 -> PWM Generator (DC-DC)/1, [D]
  Add/1 -> Saturation/1  "D"
  MPPT/1(Delta_D) -> Add/2
  Duty Cycle/1 -> Add/1

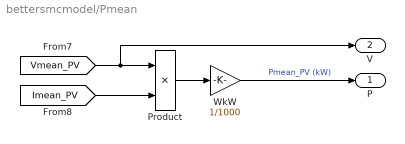
== system bettersmcmodel/Pmean ==
  Product : Product  RndMeth=Zero
  WkW : Gain  Gain=1/1000
  P : Outport
  V : Outport  Port=2
  wires:
  [Vmean_PV] -> Product/1, V/1
  Product/1 -> WkW/1
  [Imean_PV] -> Product/2
  WkW/1 -> P/1  "Pmean_PV (kW)"

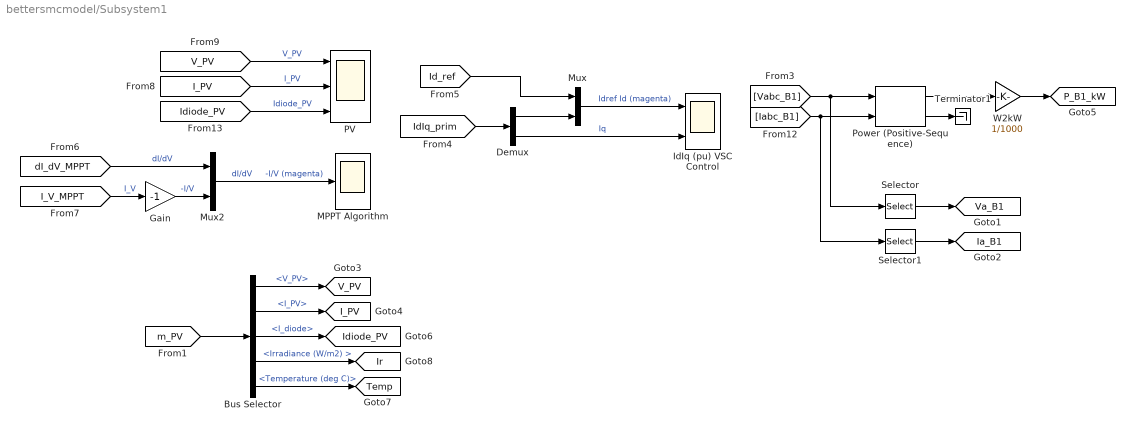
== system bettersmcmodel/Subsystem1 ==
  Bus Selector : BusSelector  OutputSignals=V_PV,I_PV,I_diode,Irradiance (W/m2) ,Temperature (deg C)
  Demux : Demux  Outputs=2
  Gain : Gain  Gain=-1
  IdIq (pu) VSC Control : Scope  NumInputPorts=2
      settings: TimeRange=2  YMin=-5~-5  YMax=5~5  Decimation=100
  MPPT Algorithm : Scope
      settings: TimeRange=2  Decimation=100
  Mux : Mux  Inputs=2
  Mux2 : Mux  Inputs=2
  PV : Scope  NumInputPorts=3
      settings: TimeRange=2  YMin=-5~-5~-5  YMax=5~5~5  Decimation=100
  Power (Positive-Sequence) : powerlib_meascontrol/Measurements/Power (Positive-Sequence)  Freq=60  Vinit=[0, 0]  Iinit=[0, 0]  Ts=Ts_Control
  Selector : Selector  InputPortWidth=3  Indices=[1]
  Selector1 : Selector  InputPortWidth=3  Indices=[1]
  Terminator1 : Terminator
  W2kW : Gain  Gain=1/1000
  tag scope: I_PV=global, Ia_B1=global, Idiode_PV=global, Ir=global, P_B1_kW=global, Temp=global, V_PV=global, Va_B1=global
  wires:
  [Vabc_B1] -> Power (Positive-Sequence)/1, Selector/1
  [Iabc_B1] -> Power (Positive-Sequence)/2, Selector1/1
  Power (Positive-Sequence)/1 -> W2kW/1
  [I_V_MPPT] -> Gain/1  "I_V"
  [IdIq_prim] -> Demux/1
  [Id_ref] -> Mux/1
  Demux/1 -> Mux/2
  Mux/1 -> IdIq (pu) VSC Control/1  "Idref Id (magenta)"
  Demux/2 -> IdIq (pu) VSC Control/2  "Iq"
  Selector/1 -> [Va_B1]
  Selector1/1 -> [Ia_B1]
  [V_PV] -> PV/1  "V_PV"
  [I_PV] -> PV/2  "I_PV"
  [Idiode_PV] -> PV/3  "Idiode_PV"
  [dI_dV_MPPT] -> Mux2/1  "dI/dV"
  Gain/1 -> Mux2/2  "-I/V"
  Mux2/1 -> MPPT Algorithm/1  "dI/dV     -I/V (magenta)"
  W2kW/1 -> [P_B1_kW]
  [m_PV] -> Bus Selector/1
  Bus Selector/1 -> [V_PV]  "<V_PV>"
  Bus Selector/2 -> [I_PV]  "<I_PV>"
  Bus Selector/4 -> [Ir]  "<Irradiance (W/m2) >"
  Bus Selector/3 -> [Idiode_PV]  "<I_diode>"
  Bus Selector/5 -> [Temp]  "<Temperature (deg C)>"
  Power (Positive-Sequence)/2 -> Terminator1/1

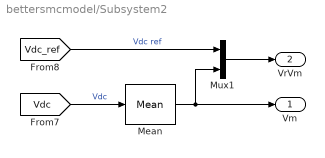
== system bettersmcmodel/Subsystem2 ==
  Mean : powerlib_meascontrol/Measurements/Mean  Freq=60  Vinit=0  Ts=Ts_Control
  Mux1 : Mux  Inputs=2
  Vm : Outport
  VrVm : Outport  Port=2
  wires:
  [Vdc_ref] -> Mux1/1  "Vdc ref"
  [Vdc] -> Mean/1  "Vdc"
  Mux1/1 -> VrVm/1
  Mean/1 -> Mux1/2, Vm/1

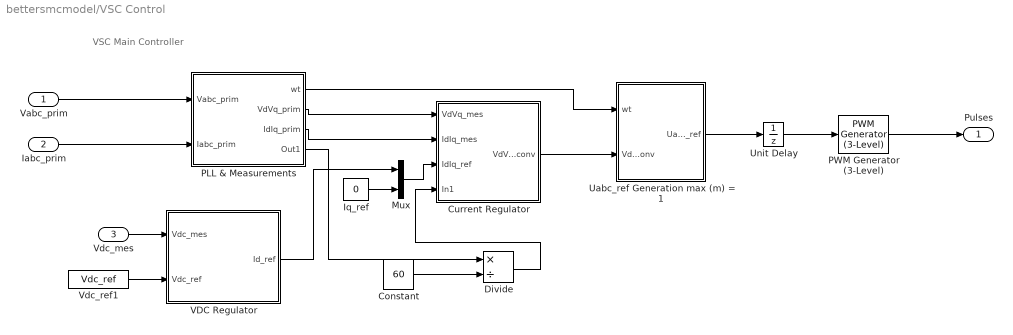
== system bettersmcmodel/VSC Control ==
  note: VSC Main Controller
  Vabc_prim : Inport  PortDimensions=3
  Iabc_prim : Inport  Port=2  PortDimensions=3
  Vdc_mes : Inport  Port=3  PortDimensions=1
  Constant : Constant  Value=60
  Current Regulator : Subsystem
  Divide : Product  Inputs=*/
  Iq_ref : Constant  Value=0
  Mux : Mux  Inputs=2
  PLL & Measurements : Subsystem
  PWM Generator (3-Level) : powerlib_meascontrol/Pulse & Signal Generators/PWM Generator (3-Level)  ModulatorType=Three-phase bridge (12 pulses)  ModulatorMode=Unsynchronized  nF=27  Fc=33*60  ModulatingSignals=off  m=0.8  Freq=60  Phase=0  Ts=Ts_Power
  Uabc_ref Generation max (m) = 1 : Subsystem
  Unit Delay : UnitDelay  SampleTime=Ts_Control
  VDC Regulator : Subsystem
  Vdc_ref1 : Constant  Value=Vdc_ref
  Pulses : Outport
  wires:
  VDC Regulator/1(Id_ref) -> Mux/1
  PLL & Measurements/1(wt) -> Uabc_ref Generation max (m) = 1/1(wt)
  Current Regulator/1(VdVq_conv) -> Uabc_ref Generation max (m) = 1/2(VdVq_conv)
  Iq_ref/1 -> Mux/2
  Mux/1 -> Current Regulator/3(IdIq_ref)
  PLL & Measurements/3(IdIq_prim) -> Current Regulator/2(IdIq_mes)
  PLL & Measurements/2(VdVq_prim) -> Current Regulator/1(VdVq_mes)
  Vdc_mes/1 -> VDC Regulator/1(Vdc_mes)
  Vabc_prim/1 -> PLL & Measurements/1(Vabc_prim)
  Iabc_prim/1 -> PLL & Measurements/2(Iabc_prim)
  Unit Delay/1 -> PWM Generator (3-Level)/1
  PWM Generator (3-Level)/1 -> Pulses/1
  Uabc_ref Generation max (m) = 1/1(Uabc_ref) -> Unit Delay/1
  Vdc_ref1/1 -> VDC Regulator/2(Vdc_ref)
  Constant/1 -> Divide/2
  PLL & Measurements/4(Out1) -> Divide/1
  Divide/1 -> Current Regulator/4(In1)

== system bettersmcmodel/info ==

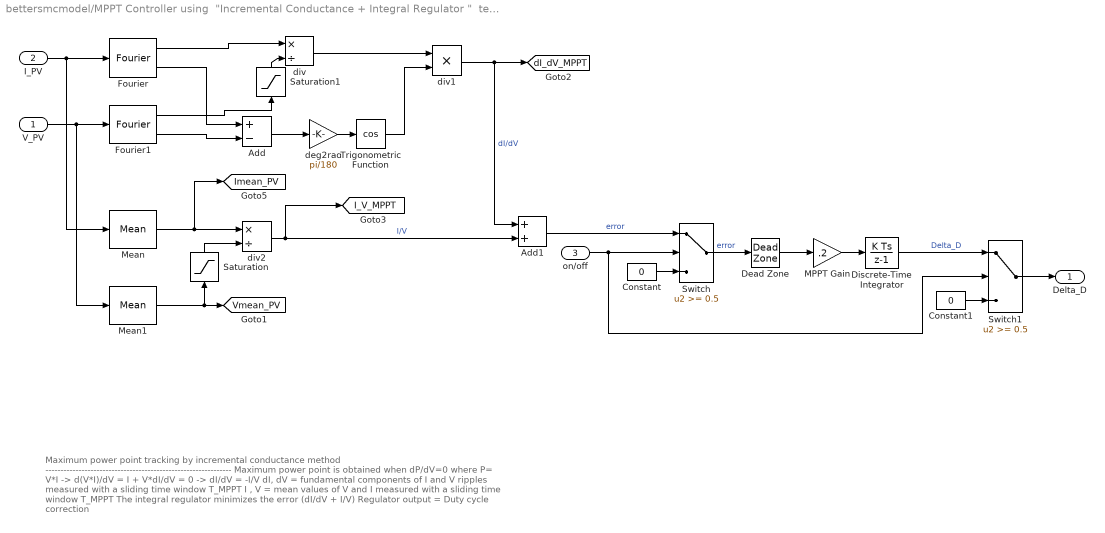
== system bettersmcmodel/MPPT Controller using  "Incremental Conductance + Integral Regulator "  technique /MPPT ==
  note: Maximum power point tracking by incremental conductance method
      | --------------------------------------------------------------
      | Maximum power point is obtained when dP/dV=0  where P= V*I
      | -> d(V*I)/dV = I + V*dI/dV = 0
      | -> dI/dV = -I/V
      |
      | dI, dV  = fundamental components of I and V ripples measured with a sliding time window T_MPPT
      | I , V   = mean values of V and I measured with a sliding time window T_MPPT
      |
      | The integral regulator minimizes the error (dI/dV + I/V)
      | Regulator output = Duty cycle correction
  V_PV : Inport
  I_PV : Inport  Port=2
  on/off : Inport  Port=3
  Add : Sum  Inputs=+-
  Add1 : Sum
  Constant : Constant  Value=0
  Constant1 : Constant  Value=0
  Dead Zone : DeadZone  LowerValue=-0.05  UpperValue=0.05  SaturateOnIntegerOverflow=on
  Discrete-Time Integrator : DiscreteIntegrator  SampleTime=Ts_Control  LimitOutput=on  UpperSaturationLimit=1  LowerSaturationLimit=-1
  Fourier : powerlib_meascontrol/Measurements/Fourier  Freq=1/T_MPPT  n=1  InInit=[0, 0]  Ts=Ts_Control
  Fourier1 : powerlib_meascontrol/Measurements/Fourier  Freq=1/T_MPPT  n=1  InInit=[0, 0]  Ts=Ts_Control
  MPPT Gain : Gain  Gain=.2
  Mean : powerlib_meascontrol/Measurements/Mean  Freq=1/T_MPPT  Vinit=0  Ts=Ts_Control
  Mean1 : powerlib_meascontrol/Measurements/Mean  Freq=1/T_MPPT  Vinit=0  Ts=Ts_Control
  Saturation : Saturate  UpperLimit=inf  LowerLimit=eps
  Saturation1 : Saturate  UpperLimit=inf  LowerLimit=eps
  Switch : Switch  Threshold=0.5
  Switch1 : Switch  Threshold=0.5
  Trigonometric Function : Trigonometry  Operator=cos
  deg2rad : Gain  Gain=pi/180
  div : Product  Inputs=*/  RndMeth=Zero
  div1 : Product  Inputs=**  RndMeth=Zero
  div2 : Product  Inputs=*/  RndMeth=Zero
  Delta_D : Outport
  tag scope: I_V_MPPT=global, Imean_PV=global, Vmean_PV=global, dI_dV_MPPT=global
  wires:
  Dead Zone/1 -> MPPT Gain/1
  Switch/1 -> Dead Zone/1  "error"
  Saturation1/1 -> div/2
  Saturation/1 -> div2/2
  Switch1/1 -> Delta_D/1
  on/off/1 -> Switch/2, Switch1/2
  Constant1/1 -> Switch1/3
  Discrete-Time Integrator/1 -> Switch1/1  "Delta_D"
  Constant/1 -> Switch/3
  MPPT Gain/1 -> Discrete-Time Integrator/1
  Add1/1 -> Switch/1  "error"
  div2/1 -> Add1/2, [I_V_MPPT]  "I/V"
  Mean1/1 -> Saturation/1, [Vmean_PV]
  Mean/1 -> div2/1, [Imean_PV]
  div1/1 -> Add1/1, [dI_dV_MPPT]  "dI/dV"
  Trigonometric Function/1 -> div1/2
  div/1 -> div1/1
  deg2rad/1 -> Trigonometric Function/1
  Add/1 -> deg2rad/1
  Fourier1/1 -> Saturation1/1
  Fourier1/2 -> Add/2
  Fourier/2 -> Add/1
  V_PV/1 -> Mean1/1, Fourier1/1
  I_PV/1 -> Mean/1, Fourier/1
  Fourier/1 -> div/1

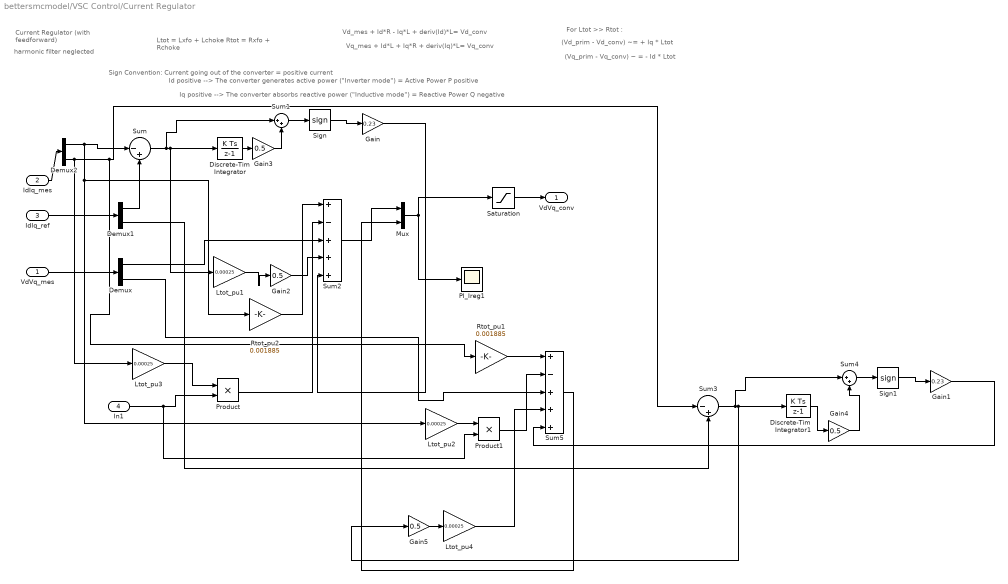
== system bettersmcmodel/VSC Control/Current Regulator ==
  note: harmonic filter neglected
  note: Vd_mes + Id*R - Iq*L + deriv(Id)*L= Vd_conv
  note: Vq_mes + Id*L + Iq*R + deriv(Iq)*L= Vq_conv
  note: Current Regulator
      | (with feedforward)
  note: Sign Convention: Current going out of the converter = positive current
  note: Iq positive --> The converter absorbs reactive power ("Inductive mode") = Reactive Power Q negative
  note: Id positive --> The converter generates active power ("Inverter mode") = Active Power P positive
  note: Ltot = Lxfo + Lchoke
      | Rtot = Rxfo + Rchoke
  note: (Vd_prim - Vd_conv) ~= + Iq * Ltot
  note: (Vq_prim - Vq_conv) ~ = - Id * Ltot
  note: For Ltot >> Rtot :
  VdVq_mes : Inport  PortDimensions=2
  IdIq_mes : Inport  Port=2  PortDimensions=2
  IdIq_ref : Inport  Port=3  PortDimensions=2
  In1 : Inport  Port=4
  Demux : Demux  Outputs=2
  Demux1 : Demux  Outputs=2
  Demux2 : Demux  Outputs=2
  Discrete-Tim Integrator : DiscreteIntegrator  InitialConditionSetting=State (most efficient)
  Discrete-Tim Integrator1 : DiscreteIntegrator  InitialConditionSetting=State (most efficient)
  Gain : Gain  Gain=0.23
  Gain1 : Gain  Gain=0.23
  Gain{2..5} (4 alike) : Gain  Gain=0.5
  Ltot_pu{1..4} (4 alike) : Gain  Gain=0.00025  SaturateOnIntegerOverflow=on  OutDataTypeStr=Inherit: Same as input  ParamDataTypeStr=Inherit: Same as input
  Mux : Mux  Inputs=2
  PI_Ireg1 : Scope
  Product : Product
  Product1 : Product
  Rtot_pu1 : Gain  Gain=0.001885  SaturateOnIntegerOverflow=on  OutDataTypeStr=Inherit: Same as input  ParamDataTypeStr=Inherit: Same as input
  Rtot_pu2 : Gain  Gain=0.001885  SaturateOnIntegerOverflow=on  OutDataTypeStr=Inherit: Same as input  ParamDataTypeStr=Inherit: Same as input
  Saturation : Saturate  UpperLimit=2  LowerLimit=-2
  Sign : Signum
  Sign1 : Signum
  Sum : Sum  Inputs=|-+
  Sum1 : Sum  Inputs=|++
  Sum2 : Sum  Inputs=+-+++
  Sum3 : Sum  Inputs=|-+
  Sum4 : Sum  Inputs=|++
  Sum5 : Sum  Inputs=+-+++
  VdVq_conv : Outport
  wires:
  IdIq_ref/1 -> Demux1/1
  IdIq_mes/1 -> Demux2/1
  Mux/1 -> Saturation/1, PI_Ireg1/1
  Saturation/1 -> VdVq_conv/1
  VdVq_mes/1 -> Demux/1
  Demux1/1 -> Sum/2
  In1/1 -> Product1/2, Product/2
  Ltot_pu3/1 -> Product/1
  Demux/1 -> Sum2/3
  Sum/1 -> Discrete-Tim Integrator/1, Ltot_pu1/1, Sum1/1
  Discrete-Tim Integrator/1 -> Gain3/1
  Sign/1 -> Gain/1
  Sum1/1 -> Sign/1
  Rtot_pu2/1 -> Sum2/1
  Product/1 -> Sum2/2
  Ltot_pu1/1 -> Gain2/1
  Gain/1 -> Sum2/5
  Sum2/1 -> Mux/1
  Ltot_pu2/1 -> Product1/1
  Demux2/1 -> Ltot_pu2/1, Rtot_pu2/1, Sum/1
  Demux/2 -> Sum5/3
  Sum3/1 -> Gain5/1, Discrete-Tim Integrator1/1, Sum4/1
  Discrete-Tim Integrator1/1 -> Gain4/1
  Sign1/1 -> Gain1/1
  Sum4/1 -> Sign1/1
  Gain1/1 -> Sum5/5
  Demux2/2 -> Ltot_pu3/1, Sum3/1, Rtot_pu1/1
  Demux1/2 -> Sum3/2
  Rtot_pu1/1 -> Sum5/1
  Product1/1 -> Sum5/2
  Ltot_pu4/1 -> Sum5/4
  Sum5/1 -> Mux/2
  Gain2/1 -> Sum2/4
  Gain3/1 -> Sum1/2
  Gain4/1 -> Sum4/2
  Gain5/1 -> Ltot_pu4/1

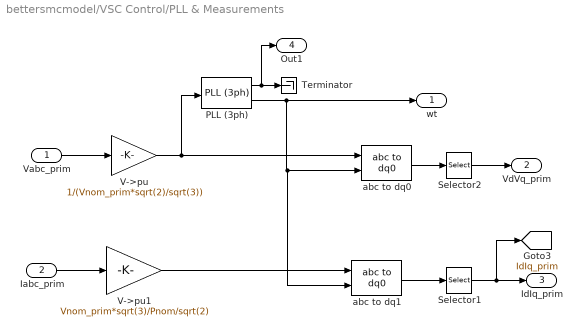
== system bettersmcmodel/VSC Control/PLL & Measurements ==
  Vabc_prim : Inport
  Iabc_prim : Inport  Port=2
  PLL (3ph) : powerlib_meascontrol/PLL/PLL (3ph)  Fmin=45  Par_Init="[-0.57  Fnom]"  ParK=[180, 3200, 1]  TcD=1e-4  MaxRateChangeFreq=12  FilterCutOffFreq=25  Ts=Ts  AGC=on
  Selector1 : Selector  InputPortWidth=3  Indices=[1 2]
  Selector2 : Selector  InputPortWidth=3  Indices=[1 2]
  Terminator : Terminator
  V->pu : Gain  Gain=1/(Vnom_prim*sqrt(2)/sqrt(3))  SaturateOnIntegerOverflow=on  OutDataTypeStr=Inherit: Same as input  ParamDataTypeStr=Inherit: Same as input
  V->pu1 : Gain  Gain=Vnom_prim*sqrt(3)/Pnom/sqrt(2)  SaturateOnIntegerOverflow=on  OutDataTypeStr=Inherit: Same as input  ParamDataTypeStr=Inherit: Same as input
  abc to dq0 : powerlib_meascontrol/Transformations/abc to dq0  Alignment=90 degrees behind phase A axis
  abc to dq1 : powerlib_meascontrol/Transformations/abc to dq0  Alignment=90 degrees behind phase A axis
  wt : Outport
  VdVq_prim : Outport  Port=2
  IdIq_prim : Outport  Port=3
  Out1 : Outport  Port=4
  tag scope: IdIq_prim=global
  wires:
  V->pu1/1 -> abc to dq1/1
  V->pu/1 -> PLL (3ph)/1, abc to dq0/1
  abc to dq1/1 -> Selector1/1
  Vabc_prim/1 -> V->pu/1
  Iabc_prim/1 -> V->pu1/1
  abc to dq0/1 -> Selector2/1
  Selector2/1 -> VdVq_prim/1
  Selector1/1 -> [IdIq_prim], IdIq_prim/1
  PLL (3ph)/2 -> wt/1, abc to dq1/2, abc to dq0/2
  PLL (3ph)/1 -> Out1/1, Terminator/1

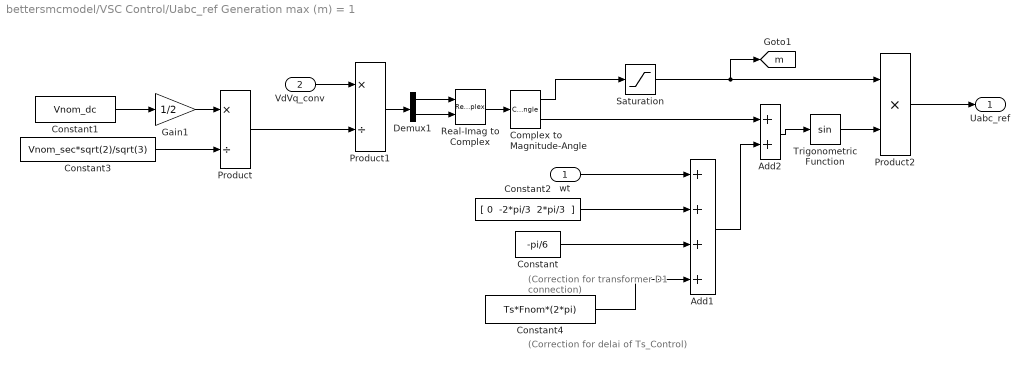
== system bettersmcmodel/VSC Control/Uabc_ref Generation max (m) = 1 ==
  note: (Correction for transformer
      |  D1 connection)
  note: (Correction for delai of Ts_Control)
  wt : Inport
  VdVq_conv : Inport  Port=2
  Add1 : Sum  Inputs=++++
  Add2 : Sum
  Complex to Magnitude-Angle : ComplexToMagnitudeAngle
  Constant : Constant  Value=-pi/6
  Constant1 : Constant  Value=Vnom_dc
  Constant2 : Constant  Value="[ 0  -2*pi/3  2*pi/3  ]"
  Constant3 : Constant  Value=Vnom_sec*sqrt(2)/sqrt(3)
  Constant4 : Constant  Value=Ts*Fnom*(2*pi)
  Demux1 : Demux  Outputs=2
  Gain1 : Gain  Gain=1/2
  Product : Product  Inputs=*/  RndMeth=Zero
  Product1 : Product  Inputs=*/  RndMeth=Zero
  Product2 : Product  Inputs=**  RndMeth=Zero
  Real-Imag to Complex : RealImagToComplex
  Saturation : Saturate  UpperLimit=1  LowerLimit=0
  Trigonometric Function : Trigonometry
  Uabc_ref : Outport
  tag scope: m=global
  wires:
  Complex to Magnitude-Angle/1 -> Saturation/1
  Constant1/1 -> Gain1/1
  VdVq_conv/1 -> Product1/1
  Product1/1 -> Demux1/1
  Gain1/1 -> Product/1
  Real-Imag to Complex/1 -> Complex to Magnitude-Angle/1
  Demux1/1 -> Real-Imag to Complex/1
  Demux1/2 -> Real-Imag to Complex/2
  Constant2/1 -> Add1/2
  Constant/1 -> Add1/3
  Constant3/1 -> Product/2
  Product/1 -> Product1/2
  Complex to Magnitude-Angle/2 -> Add2/1
  Add1/1 -> Add2/2
  Add2/1 -> Trigonometric Function/1
  Saturation/1 -> [m], Product2/1
  Trigonometric Function/1 -> Product2/2
  Product2/1 -> Uabc_ref/1
  wt/1 -> Add1/1
  Constant4/1 -> Add1/4
